simulink model "With-Attack"  (R2018b)
settings: Solver=VariableStepAuto  StartTime=0.0  StopTime=10.0  RelTol=1e-3
undefined symbols (not defined in the file or in its folder): sigbuilder_block
settings Model: Creator=lenovo  LastModifiedBy=lenovo

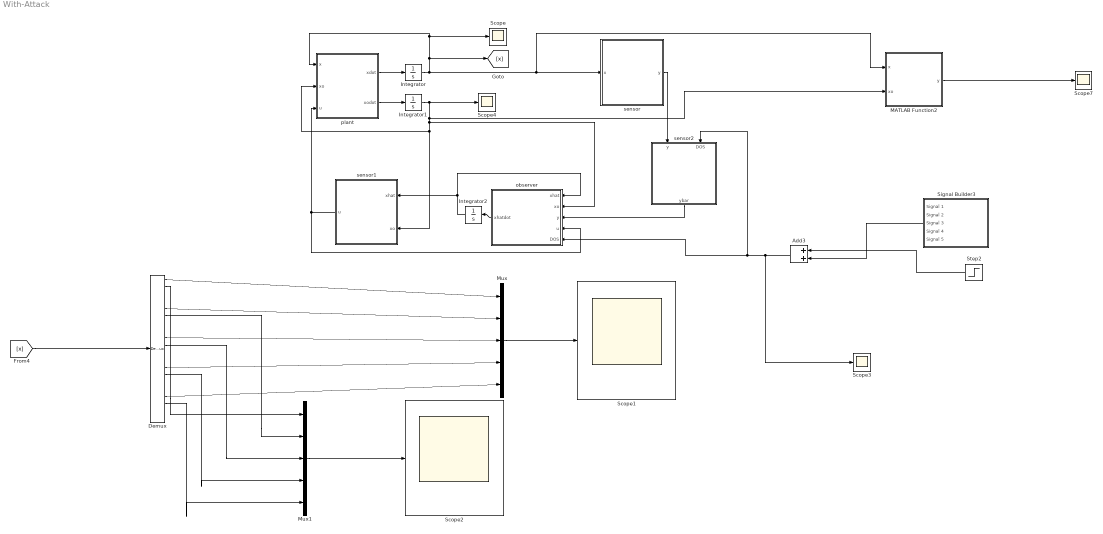
== system With-Attack ==
  Add3 : Sum
  Demux : Demux  Outputs=20
  Integrator : Integrator  InitialCondition=[-10;-9;-8;-7;-6;5;-4;-3;-2;-1;1;2;3;4;5;6;7;8;9;10]
  Integrator1 : Integrator  InitialCondition=[-5;1;3;-15]
  Integrator2 : Integrator  InitialCondition=[-10;-9;-8;-7;-6;5;-4;-3;-2;-1;1;2;3;4;5;6;7;8;9;10]
  MATLAB Function2 : MATLAB Function  TreatAsAtomicUnit=on
  Mux : Mux  Inputs=5
  Mux1 : Mux  Inputs=5
  Scope{,1..4,7} (6 alike) : Scope
  Signal Builder3 : Subsystem  Tag=STV Subsys  LoadFcn=sigbuilder_block('load');  StartFcn=sigbuilder_block('start');  StopFcn=sigbuilder_block('stop');  ClipboardFcn=sigbuilder_block('clipboard');  mask(Sigbuilder block){tuvar=[0:10]}
      mask help: Simulink:masks:SigbuilderBlock_MD
      mask init:
      | if ~strcmp(get_param(bdroot(gcbh),'SimulationStatus'),'stopped') tuvar = sigbuilder_block('maskInit'); end
      settings: CopyFcn=sigbuilder_block('copy');  DeleteFcn=sigbuilder_block('delete');  ModelCloseFcn=sigbuilder_block('modelClose');  PreSaveFcn=sigbuilder_block('preSave');  PauseFcn=sigbuilder_block('pause');  ContinueFcn=sigbuilder_block('continue');  NameChangeFcn=sigbuilder_block('namechange');  OpenFcn=sigbuilder_block('open',[5.4 30 1141.2 522.6 ]);  CloseFcn=sigbuilder_block('close');
      mask Display: plot(0, 0, 100, 100,[2, 2, 32, 32, 2], [68, 8, 8, 68, 68],[32, 2], [38, 38], [32, 19, 2],[53, 60, 44], [32, 17, 17, 2],[16, 16, 31, 31]);txt = getActiveGroup(gcbh);text(2, 100, txt,'verticalAlignment', 'top');
  Step2 : Step  After=-1  SampleTime=10
  observer : MATLAB Function  TreatAsAtomicUnit=on
  plant : MATLAB Function  TreatAsAtomicUnit=on
  sensor : MATLAB Function  TreatAsAtomicUnit=on
  sensor1 : MATLAB Function  TreatAsAtomicUnit=on
  sensor2 : MATLAB Function  TreatAsAtomicUnit=on
  wires:
  sensor2/1(ybar) -> observer/3(y)
  sensor1/1(u) -> plant/3(u), observer/4(u)
  observer/1(xhatdot) -> Integrator2/1
  sensor/1(y) -> sensor2/1(y)
  plant/1(xdot) -> Integrator/1
  plant/2(xodot) -> Integrator1/1
  Integrator2/1 -> observer/1(xhat), sensor1/1(xhat)
  Integrator/1 -> [x], Scope/1, plant/1(x), MATLAB Function2/1(x), sensor/1(x)
  Integrator1/1 -> Scope4/1, MATLAB Function2/2(xo), observer/2(xo), sensor1/2(xo), plant/2(xo)
  MATLAB Function2/1(y) -> Scope7/1
  Add3/1 -> Scope3/1, observer/5(DOS), sensor2/2(DOS)
  Signal Builder3/3(Signal 3) -> Add3/2
  Step2/1 -> Add3/1
  Demux/5 -> Mux/2
  Demux/17 -> Mux/5
  Mux/1 -> Scope1/1
  Demux/13 -> Mux/4
  Demux/1 -> Mux/1
  [x] -> Demux/1
  Demux/14 -> Mux1/4
  Demux/9 -> Mux/3
  Demux/6 -> Mux1/2
  Demux/2 -> Mux1/1
  Demux/10 -> Mux1/3
  Mux1/1 -> Scope2/1
  Demux/18 -> Mux1/5

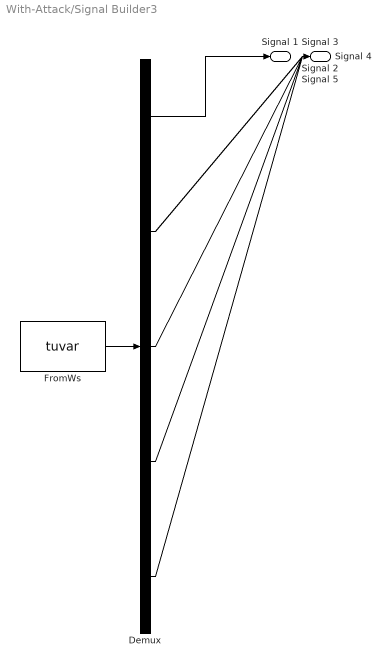
== system With-Attack/Signal Builder3 ==
  Demux : Demux  Tag=STV Demux  Outputs=5
  FromWs : FromWorkspace  Tag=STV FromWs  VariableName=tuvar  SampleTime=0
      SigBuilderData=|
      | common.afterFinalStr = 'Extrapolate'
      | common.sampleTime = 0
      | dataSet.timeRange = [0 10]
      | dataSet.name = 'Group 1'
      | sbobj.Groups.Name = 'Group 1'
      | sbobj.Groups.Signals(1).Name = 'Signal 1'
      | sbobj.Groups.Signals(1).XData = [0 4 4 6 6 10]
      | sbobj.Groups.Signals(1).YData = [0 0 1 1 0 0]
      | sbobj.Groups.Signals(2).Name = 'Signal 2'
      | sbobj.Groups.Signals(2).XData = [0 0.125 0.125 0.25 0.25 0.375 0.375 0.5 0.5 0.625 0.625 0.75 0.75 0.875 0.875 1 1 1.125 1.125 1.25 1.25 1.375 1.375 1.5 1.5 1.625 1.625 1.75 1.75 1.875 1.875 2 2 2.125 2.125 2.25 2.25 2.375 2.375 2.5 2.5 2.625 2.625 2.75 2.75 2.875 2.875 3 3 3.125 3.125 3.25 3.25 3.375 3.375 3.5 3.5 3.625 3.625 3.75 3.75 3.875 3.875 4 4 4.125 4.125 4.25 4.25 4.375 4.375 4.5 4.5 4.625 4.625 4.75 4.75 4.875 4.875 5 5 5.125 5.125 5.25 5.25 5.375 5.375 5.5 5.5 5.625 5.625 5.75 5.75 5.875 5.875 6 6 6.125 6.125 6.25 6.25 6.375 6.375 6.5 6.5 6.625 6.625 6.75 6.75 6.875 6.875 7 7 7.125 7.125 7.25 7.25 7.375 7.375 7.5 7.5 7.625 7.625 7.75 7.75 7.875 7.875 8 8 8.125 8.125 8.25 8.25 8.375 8.375 8.5 8.5 8.625 8.625 8.75 8.75 8.875 8.875 9 9 9.125 9.125 9.25 9.25 9.375 9.375 9.5 9.5 9.625 9.625 9.75 9.75 9.875 9.875 10]
      | sbobj.Groups.Signals(2).YData = [1 1 -1 -1 1 1 -1 -1 1 1 -1 -1 1 1 -1 -1 1 1 -1 -1 1 1 -1 -1 1 1 -1 -1 1 1 -1 -1 1 1 -1 -1 1 1 -1 -1 1 1 -1 -1 1 1 -1 -1 1 1 -1 -1 1 1 -1 -1 1 1 -1 -1 1 1 -1 -1 1 1 -1 -1 1 1 -1 -1 1 1 -1 -1 1 1 -1 -1 1 1 -1 -1 1 1 -1 -1 1 1 -1 -1 1 1 -1 -1 1 1 -1 -1 1 1 -1 -1 1 1 -1 -1 1 1 -1 -1 1 1 -1 -1 1 1 -1 -1 1 1 -1 -1 1 1 -1 -1 1 1 -1 -1 1 1 -1 -1 1 1 -1 -1 1 1 -1 -1 1 1 -1 -1 1 1 -1 -1 1 1 -1 -1 1 1 -1 -1]
      | sbobj.Groups.Signals(3).Name = 'Signal 3'
      | sbobj.Groups.Signals(3).XData = [0 0.16 0.333333333333 0.4 0.4 0.46 0.46 0.833333333333 1 1.005 1.005 1.3 1.3 1.8 1.8 1.9 1.9 2.4 2.4 2.55 2.55 2.625 2.785 2.83333333333 3 3.2 3.2 3.4 3.4 3.5 3.66666666667 3.83333333333 4 4 4.17 4.17 4.33333333333 4.5 4.8 4.8 4.85 4.85 5 5.16666666667 5.33333333333 5.33333333333 5.5 5.5 5.66666666667 5.83333333333 5.83333333333 6 6 6.16666666667 6.33333333333 6.5 6.5 6.66666666667 6.66666666667 6.83333333333 7 7 7.16666666667 7.16666666667 7.33333333333 7.5 7.66666666667 7.83333333333 7.83333333333 8 8 8.16666666667 8.33333333333 8.5 8.5 8.66666666667 8.66666666667 8.83333333333 9 9.16666666667 9.33333333333 9.33333333333 9.5 9.5 9.66666666667 9.83333333333 10]
      | sbobj.Groups.Signals(3).YData = [1 1 1 1 0 0 1 1 1 1 0 0 1 1 0 0 1 1 0 0 1 1 1 1 1 1 0 0 1 1 1 1 1 0 0 1 1 1 1 0 0 1 1 1 1 0 0 1 1 1 0 0 1 1 1 1 0 0 1 1 1 0.005 0.005 1 1 1 1 1 0 0 1 1 1 1 0 0 1 1 1 1 1 0 0 1 1 1 1]
      | sbobj.Groups.Signals(4).Name = 'Signal 4'
      | sbobj.Groups.Signals(4).XData = [0 5 5 10]
      | sbobj.Groups.Signals(4).YData = [0 0 1 1]
      | sbobj.Groups.Signals(5).Name = 'Signal 5'
      | sbobj.Groups.Signals(5).XData = [0 0.45 0.45 0.5 0.5 0.95 0.95 1 1 1.45 1.45 1.5 1.5 1.95 1.95 2 2 2.45 2.45 2.5 2.5 2.95 2.95 3 3 3.45 3.45 3.5 3.5 3.95 3.95 4 4 4.45 4.45 4.5 4.5 4.95 4.95 5 5 5.45 5.45 5.5 5.5 5.95 5.95 6 6 6.45 6.45 6.5 6.5 6.95 6.95 7 7 7.45 7.45 7.5 7.5 7.95 7.95 8 8 8.45 8.45 8.5 8.5 8.95 8.95 9 9 9.45 9.45 9.5 9.5 9.95 9.95 10]
      | sbobj.Groups.Signals(5).YData = [1 1 0 0 1 1 0 0 1 1 0 0 1 1 0 0 1 1 0 0 1 1 0 0 1 1 0 0 1 1 0 0 1 1 0 0 1 1 0 0 1 1 0 0 1 1 0 0 1 1 0 0 1 1 0 0 1 1 0 0 1 1 0 0 1 1 0 0 1 1 0 0 1 1 0 0 0.995 0.995 0 0]
  Signal 1 : Outport  Tag=STV Outport
  Signal 2 : Outport  Tag=STV Outport  Port=2
  Signal 3 : Outport  Tag=STV Outport  Port=3
  Signal 4 : Outport  Tag=STV Outport  Port=4
  Signal 5 : Outport  Tag=STV Outport  Port=5
  wires:
  Demux/1 -> Signal 1/1
  FromWs/1 -> Demux/1
  Demux/2 -> Signal 2/1
  Demux/3 -> Signal 3/1
  Demux/4 -> Signal 4/1
  Demux/5 -> Signal 5/1

== matlab function With-Attack/observer ==
  data: xhat input; xhatdot output; xo input; y input; u input; DOS input
function xhatdot = fcn(xhat,xo,y,u,DOS)
A=[0 1 0 0;-48.6 -1.26 48.6 0;0 0 0 10; 1.95 0 -1.95 0];
B=[0;21.6;0;0];
C=[1 0 1 -1;0 1 0 0];
teta=5;
H=[3.0849 0.6931;2.4258 34.9384;7.0235 3.5334;.54 1.8007];
R=[-0.9886 0.0381;0 -1; -1.0405 .0402;-1.0291 0.0783];

%Lo=[0 0 0 0 0 0;-1 2-DOS 0 0 0 -1+DOS;-1+DOS -1 2-DOS 0 0 0;0 -1+DOS 0 1-DOS 0 0;0 0 -1 0 1 0;0 0 -1+DOS -1 -1 3-DOS];
% L=[0 0 0 0 0 0;-1 2 0 0 0 -1;-1 -1 2 0 0 0;0 -1 0 1 0 0;0 0 -1 0 1 0;0 0 -1 -1 -1 3];

L=[ 2 0 0 0 -1; -1 2 0 0 0; -1 0 1 0 0; 0 -1 0 1 0; 0 -1 -1 -1 3];
N=5;
A0=kron(eye(N),A);
z2=kron(L,H*C);
B0=kron(eye(N),B);
xhatdot= A0*xhat+B0*u+teta*(y-z2*xhat);

== matlab function With-Attack/plant ==
  data: x input; xdot output; xo input; xodot output; u input
function [xdot,xodot] = fcn(x,xo,u)
A=[0 1 0 0;-48.6 -1.26 48.6 0;0 0 0 10; 1.95 0 -1.95 0];
B=[0;21.6;0;0];
c=2;
K=[79.1094 5.2218 -29.6598 163.9093];
%Lo=[0 0 0 0 0 0;-1 2-DOS 0 0 0 -1+DOS;-1+DOS -1 2-DOS 0 0 0;0 -1+DOS 0 1-DOS 0 0;0 0 -1 0 1 0;0 0 -1+DOS -1 -1 3-DOS];
Lu=[-1 2 0 0 0 -1;-1 -1 2 0 0 0;0 -1 0 1 0 0;0 0 -1 0 1 0;0 0 -1 -1 -1 3];
N=5;
A0=kron(eye(N),A);
z1=kron(Lu,B*K);
B0=kron(eye(N),B);
xodot =A*xo;
xdot=A0*x+B0*u;

== matlab function With-Attack/sensor1 ==
  data: xhat input; u output; xo input
function u  = fcn(xhat,xo)
c=2;
Lu=[-1 2 0 0 0 -1;-1 -1 2 0 0 0;0 -1 0 1 0 0;0 0 -1 0 1 0;0 0 -1 -1 -1 3];
K=[1.1926    0.4512   -0.9407    1.5229];
z1=kron(Lu,K);
u=-c*z1*[xo;xhat];

== matlab function With-Attack/sensor ==
  data: x input; y output
function y  = fcn(x)
C=[1 0 1 -1;0 1 0 0];
N=5;
C0=kron(eye(N),C);
y=C0*x;

== matlab function With-Attack/sensor2 ==
  data: y input; ybar output; DOS input
function ybar  = fcn(y,DOS)
Lo=[ 2-DOS 0 0 0 -1+DOS; -1 2-DOS 0 0 0; -1+DOS 0 1-DOS 0 0; 0 -1 0 1 0; 0 -1+DOS -1 -1 3-DOS];
H=[3.0849 0.6931;2.4258 34.9384;7.0235 3.5334;.54 1.8007];
L=[ 2 0 0 0 -1; -1 2 0 0 0; -1 0 1 0 0; 0 -1 0 1 0; 0 -1 -1 -1 3];
ybar=kron(Lo,H)*y;

== matlab function With-Attack/MATLAB Function2 ==
  data: x input; y output; xo input
function y = fcn(x,xo)
y=norm(kron(ones(5,1),xo)-x);
